simulink model "joint_space_trajectory_control_incomplete"  (R2022b)
settings: Solver=FixedStepDiscrete  StartTime=0.0  StopTime=inf  FixedStep=0.001  RelTol=1e-3  EnableMultiTasking=on
PreLoadFcn:
  | demos_common_configs();
  | 
  | collision_behavior = ones(1,52)*100;
undefined symbols (not defined in the file): ddQ2_desired, ddQ4_desired, dQ2_desired, dQ4_desired, Q2_desired, Q4_desired, q_init, T
libraries: franka_simulink_library_misc x5, franka_simulink_library x3
settings Model: SimulationMode=external  ExtModeTrigDuration=10000  Creator=vasi_ko  LastModifiedBy=s2ajami
settings SolverCC: AlgebraicLoopSolver=TrustRegion
settings DataIOCC: LimitDataPoints=on  SaveFormat=Array  ReturnWorkspaceOutputs=off
settings OptimizationCC: EnhancedBackFolding=on  PassReuseOutputArgsAs=Individual arguments  ZeroExternalMemoryAtStartup=off  ZeroInternalMemoryAtStartup=off  OptimizeBlockOrder=speed  DifferentSizesBufferReuse=on  OptimizationCustomize=off  EfficientTunableParamExpr=on
settings DebuggingCC: SolverPrmCheckMsg=warning  ParameterTunabilityLossMsg=error  UnconnectedInputMsg=warning  UnconnectedOutputMsg=warning  UnconnectedLineMsg=warning  SFUnexpectedBacktrackingDiag=warning  SFNoUnconditionalDefaultTransitionDiag=warning  SFExecutionAtInitializationDiag=none  SFMachineParentedDataDiag=warning  ArithmeticOperatorsInVariantConditions=warning
settings HardwareCC: ProdBitPerLong=64  ProdHWDeviceType=Intel->x86-64 (Linux 64)  TargetBitPerPointer=64  TargetBitPerSizeT=64  TargetBitPerPtrDiffT=64  TargetLongLongMode=on  TargetIntDivRoundTo=Zero  TargetEndianess=LittleEndian  TargetWordSize=64  TargetHWDeviceType=MATLAB Host
settings ModelReferenceCC: EnableRefExpFcnMdlSchedulingChecks=on  PropagateSignalLabelsOutOfModel=off
settings SFSimCC: SimUseLocalCustomCode=off  MATLABDynamicMemAlloc=off  CustomCodeUndefinedFunction=UseInterfaceOnly  SimTargetLang=C++
settings RTWCC: Description=Embedded Coder  SystemTargetFile=franka_emika_panda.tlc  GenCodeOnly=on  TemplateMakefile=ert_default_tmf  RTWVerbose=off  RTWUseLocalCustomCode=off  Toolchain=Franka Simulink | gmake (64-bit linux)  BuildConfiguration=Faster Runs  TargetLang=C++  DLArmComputeVersion=19.05
settings CodeAppCC: ForceParamTrailComments=on  IgnoreCustomStorageClasses=off  OperatorAnnotations=on  SimulinkDataObjDesc=on  SFDataObjDesc=on  InsertBlockDesc=on
settings STFCustomTargetCC: TargetLangStandard=C99 (ISO)  MultiwordLength=256  GenerateSampleERTMain=on  ModelReferenceCompliant=off  CombineOutputUpdateFcns=on  ERTCustomFileBanners=on  SupportNonInlinedSFcns=off  RemoveResetFunc=on  MATLABClassNameForMDSCustomization=Simulink.SoftwareTarget.ERTCustomization  CPPClassGenCompliant=on  UseToolchainInfoCompliant=on  SystemTargetFile=franka_emika_panda.tlc
settings ERTTargetCC: TargetLangStandard=C99 (ISO)  GenerateSampleERTMain=on  ModelReferenceCompliant=off  ParMdlRefBuildCompliant=off  CompOptLevelCompliant=off  ConcurrentExecutionCompliant=off  SupportContinuousTime=on  ModelStepFunctionPrototypeControlCompliant=off  ExtMode=on  ExtModeMexArgs='129.97.71.26' 0 17725  ERTCustomFileTemplate=franka_emika_panda_file_process.tlc
settings ConfigComp: CovMetricSettings=dw  CovSaveCumulativeToWorkspaceVar=on  CovSaveSingleToWorkspaceVar=on  CovExternalEMLEnable=off  CovSFcnEnable=off

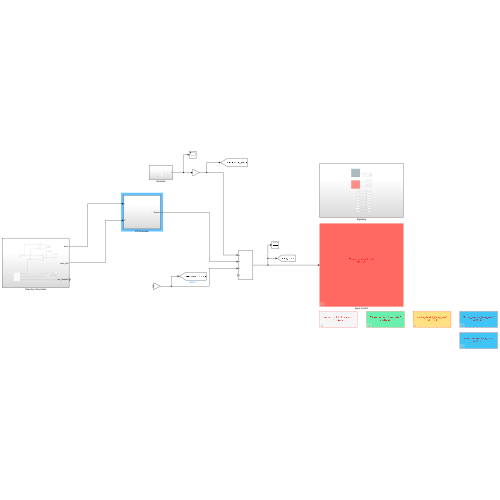
[thumbnail: Simulink's stored preview of the top-level diagram]
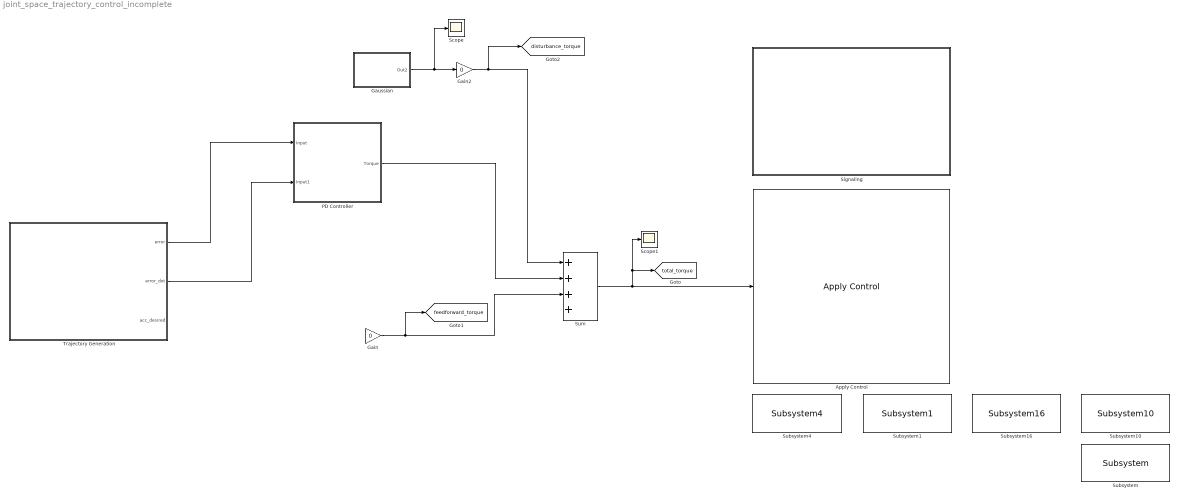
== system joint_space_trajectory_control_incomplete ==
  Apply Control : franka_simulink_library/Apply Control  robot_ip=robot_ip  gripper_attached=off  control_mode=Torque Control  controller_choice=Joint Impedance Controller  elbow_control=on  collision_thresholds=100*ones(1,52)  joint_impedance=joint_impedance  cartesian_impedance=cartesian_impedance  load_inertia=load_inertia  EE_T_K=EE_T_K  init_joint_configuration_req=on  init_joint_configuration=[0, -pi/4, 0, -3 * pi/4, 0, pi/2, pi/4]
  Gain : Gain  Gain=0
  Gain2 : Gain  Gain=0
  Gaussian : Subsystem
  PD Controller : Subsystem
  Scope : Scope
  Scope1 : Scope
  Signaling : Subsystem
  Subsystem : franka_simulink_library_misc/Subsystem  SystemSampleTime=-1  VariantActivationTime=update diagram  Latency=0  AutoFrameSizeCalculation=off
  Subsystem1 : franka_simulink_library_misc/Subsystem1  SystemSampleTime=-1  VariantActivationTime=update diagram  Latency=0  AutoFrameSizeCalculation=off
  Subsystem10 : franka_simulink_library_misc/Subsystem10  SystemSampleTime=-1  VariantActivationTime=update diagram  Latency=0  AutoFrameSizeCalculation=off
  Subsystem16 : franka_simulink_library_misc/Subsystem16  SystemSampleTime=-1  VariantActivationTime=update diagram  Latency=0  AutoFrameSizeCalculation=off
  Subsystem4 : franka_simulink_library_misc/Subsystem4  SystemSampleTime=-1  VariantActivationTime=update diagram  Latency=0  AutoFrameSizeCalculation=off
  Sum : Sum  Inputs=++++
  Trajectory Generation : Subsystem
  tag scope: disturbance_torque=global, feedforward_torque=global, total_torque=global
  wires:
  Sum/1 -> Scope1/1, [total_torque], Apply Control/1
  Trajectory Generation/1(error) -> PD Controller/1(Input)
  Trajectory Generation/2(error_dot) -> PD Controller/2(Input1)
  PD Controller/1(Torque) -> Sum/2
  Gain/1 -> [feedforward_torque], Sum/3
  Gain2/1 -> [disturbance_torque], Sum/1
  Gaussian/1(Out2) -> Scope/1, Gain2/1

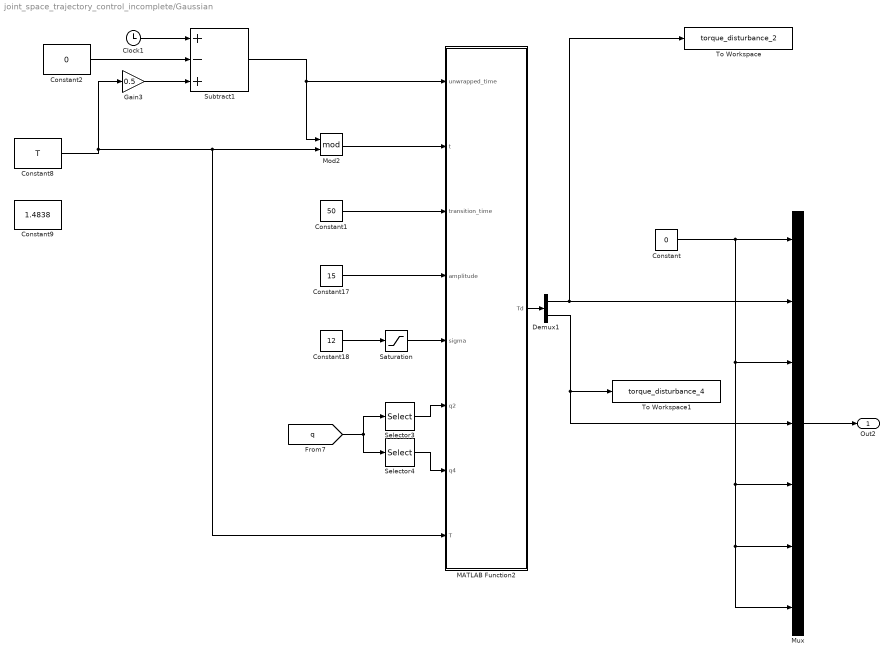
== system joint_space_trajectory_control_incomplete/Gaussian ==
  Clock1 : Clock
  Constant : Constant  Value=0
  Constant1 : Constant  Value=50
  Constant17 : Constant  Value=15
  Constant18 : Constant  Value=12
  Constant2 : Constant  Value=0
  Constant8 : Constant  Value=T
  Constant9 : Constant  Value=1.4838
  Demux1 : Demux  Outputs=2
  Gain3 : Gain  Gain=0.5
  MATLAB Function2 : MATLAB Function  TreatAsAtomicUnit=on
  Mod2 : Math  Operator=mod
  Mux : Mux  Inputs=7
  Saturation : Saturate  UpperLimit=inf  LowerLimit=12
  Selector3 : Selector  InputPortWidth=7  IndexOptions=Index vector (dialog)  Indices=[2]  OutputSizes=1
  Selector4 : Selector  InputPortWidth=7  IndexOptions=Index vector (dialog)  Indices=[4]  OutputSizes=1
  Subtract1 : Sum  Inputs=+-+
  To Workspace : ToWorkspace  VariableName=torque_disturbance_2  SaveFormat=Structure With Time  SampleTime=-1
  To Workspace1 : ToWorkspace  VariableName=torque_disturbance_4  SaveFormat=Structure With Time  SampleTime=-1
  Out2 : Outport
  wires:
  Mux/1 -> Out2/1
  Constant/1 -> Mux/3, Mux/5, Mux/6, Mux/7, Mux/1
  Gain3/1 -> Subtract1/3
  Constant17/1 -> MATLAB Function2/4(amplitude)
  Constant18/1 -> Saturation/1
  Saturation/1 -> MATLAB Function2/5(sigma)
  Clock1/1 -> Subtract1/1
  MATLAB Function2/1(Td) -> Demux1/1
  Demux1/1 -> Mux/2, To Workspace/1
  Demux1/2 -> Mux/4, To Workspace1/1
  Constant8/1 -> MATLAB Function2/8(T), Mod2/2, Gain3/1
  Mod2/1 -> MATLAB Function2/2(t)
  Subtract1/1 -> MATLAB Function2/1(unwrapped_time), Mod2/1
  Constant1/1 -> MATLAB Function2/3(transition_time)
  Constant2/1 -> Subtract1/2
  Selector3/1 -> MATLAB Function2/6(q2)
  Selector4/1 -> MATLAB Function2/7(q4)
  [q] -> Selector3/1, Selector4/1

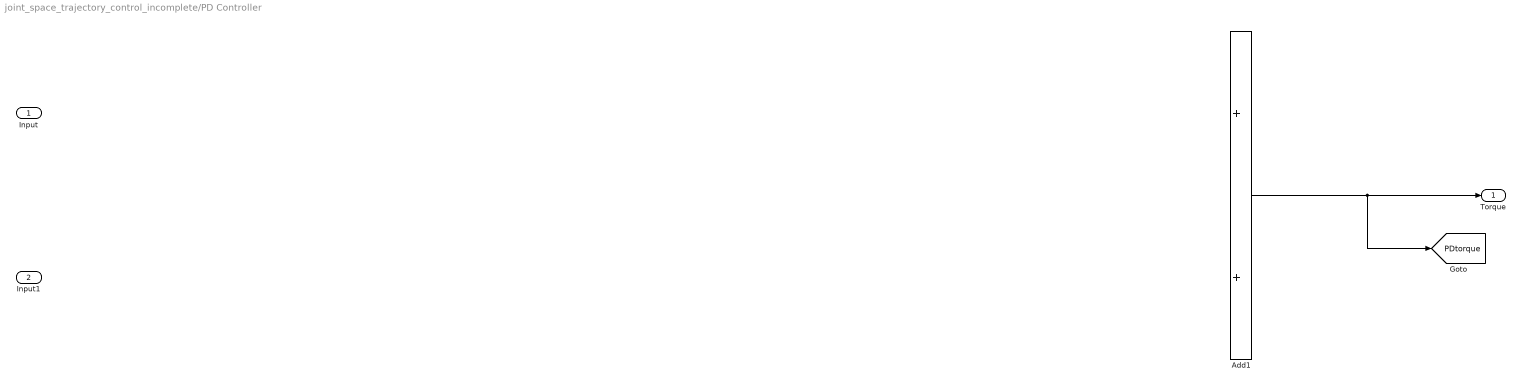
== system joint_space_trajectory_control_incomplete/PD Controller ==
  Input : Inport
  Input1 : Inport  Port=2
  Add1 : Sum
  Torque : Outport
  tag scope: PDtorque=global
  wires:
  Add1/1 -> [PDtorque], Torque/1

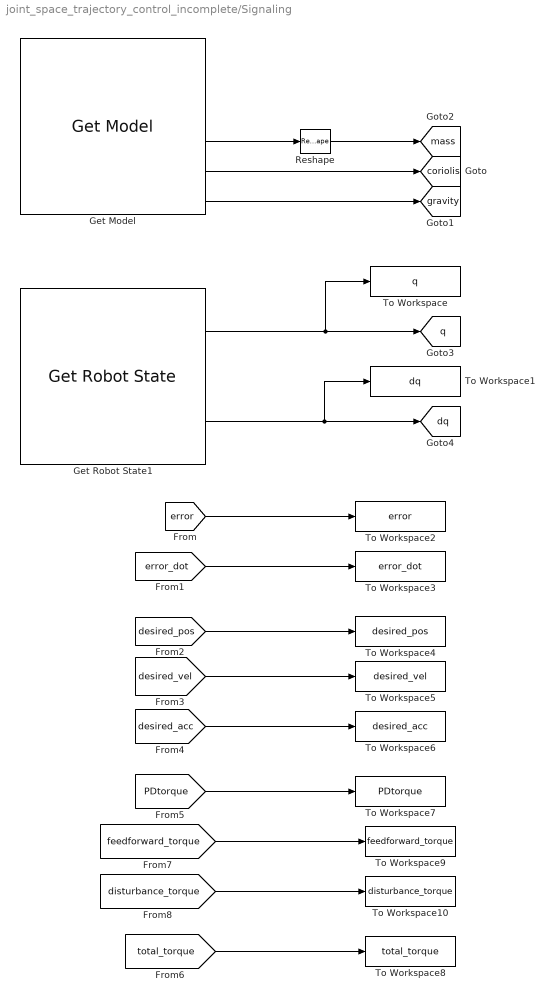
== system joint_space_trajectory_control_incomplete/Signaling ==
  Get Model : franka_simulink_library/Get Model  robot_ip=robot_ip
  Get Robot State1 : franka_simulink_library/Get Robot State  robot_ip=robot_ip  signals_requested='q dq'
  Reshape : Reshape  OutputDimensionality=Customize  OutputDimensions=[7,7]
  To Workspace : ToWorkspace  VariableName=q  SaveFormat=Structure With Time  SampleTime=-1
  To Workspace1 : ToWorkspace  VariableName=dq  SaveFormat=Structure With Time  SampleTime=-1
  To Workspace10 : ToWorkspace  VariableName=disturbance_torque  SaveFormat=Structure With Time  SampleTime=-1
  To Workspace2 : ToWorkspace  VariableName=error  SaveFormat=Structure With Time  SampleTime=-1
  To Workspace3 : ToWorkspace  VariableName=error_dot  SaveFormat=Structure With Time  SampleTime=-1
  To Workspace4 : ToWorkspace  VariableName=desired_pos  SaveFormat=Structure With Time  SampleTime=-1
  To Workspace5 : ToWorkspace  VariableName=desired_vel  SaveFormat=Structure With Time  SampleTime=-1
  To Workspace6 : ToWorkspace  VariableName=desired_acc  SaveFormat=Structure With Time  SampleTime=-1
  To Workspace7 : ToWorkspace  VariableName=PDtorque  SaveFormat=Structure With Time  SampleTime=-1
  To Workspace8 : ToWorkspace  VariableName=total_torque  SaveFormat=Structure With Time  SampleTime=-1
  To Workspace9 : ToWorkspace  VariableName=feedforward_torque  SaveFormat=Structure With Time  SampleTime=-1
  tag scope: coriolis=global, dq=global, gravity=global, mass=global, q=global
  wires:
  Get Model/5 -> [coriolis]
  Get Model/6 -> [gravity]
  Get Model/4 -> Reshape/1
  Get Robot State1/1 -> To Workspace/1, [q]
  Get Robot State1/2 -> To Workspace1/1, [dq]
  [desired_acc] -> To Workspace6/1
  [desired_vel] -> To Workspace5/1
  [desired_pos] -> To Workspace4/1
  [error_dot] -> To Workspace3/1
  [error] -> To Workspace2/1
  [PDtorque] -> To Workspace7/1
  [total_torque] -> To Workspace8/1
  Reshape/1 -> [mass]
  [feedforward_torque] -> To Workspace9/1
  [disturbance_torque] -> To Workspace10/1

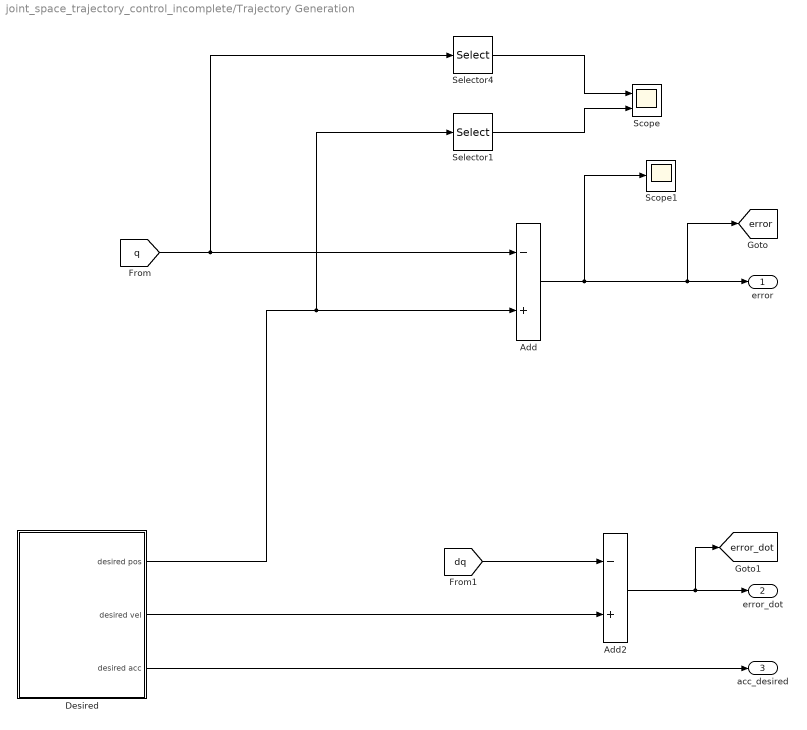
== system joint_space_trajectory_control_incomplete/Trajectory Generation ==
  Add : Sum  Inputs=-+
  Add2 : Sum  Inputs=-+
  Desired : Subsystem
  Scope : Scope  NumInputPorts=2
  Scope1 : Scope
  Selector1 : Selector  InputPortWidth=7  IndexOptions=Index vector (dialog)  Indices=[6]  OutputSizes=1
  Selector4 : Selector  InputPortWidth=7  IndexOptions=Index vector (dialog)  Indices=[6]  OutputSizes=1
  error : Outport
  error_dot : Outport  Port=2
  acc_desired : Outport  Port=3
  tag scope: error=global, error_dot=global
  wires:
  Desired/2(desired vel) -> Add2/2
  Desired/1(desired pos) -> Selector1/1, Add/2
  Add/1 -> Scope1/1, error/1, [error]
  Add2/1 -> [error_dot], error_dot/1
  Desired/3(desired acc) -> acc_desired/1
  [dq] -> Add2/1
  Selector4/1 -> Scope/1
  Selector1/1 -> Scope/2
  [q] -> Selector4/1, Add/1

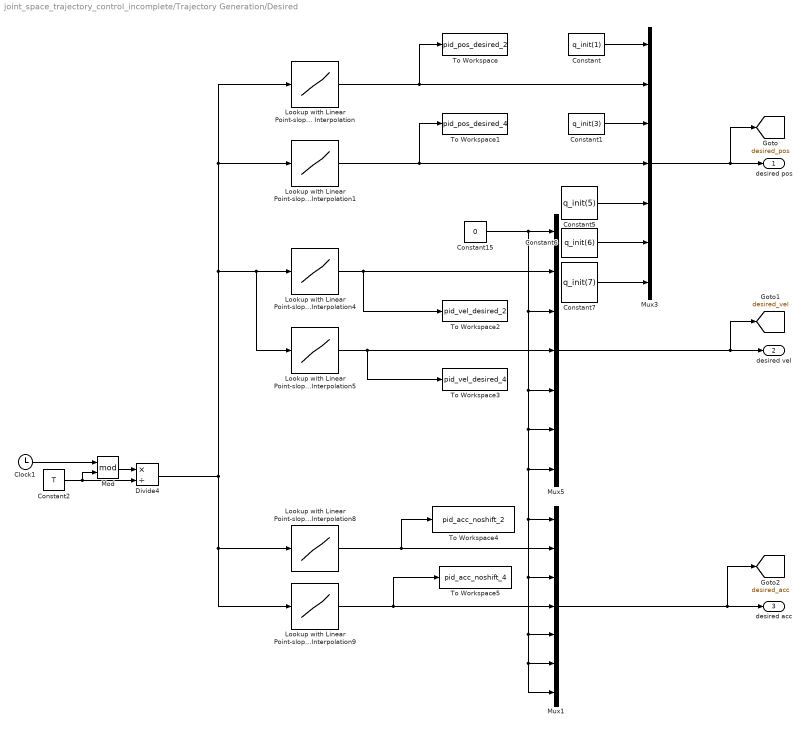
== system joint_space_trajectory_control_incomplete/Trajectory Generation/Desired ==
  Clock1 : Clock
  Constant : Constant  Value=q_init(1)
  Constant1 : Constant  Value=q_init(3)
  Constant15 : Constant  Value=0
  Constant2 : Constant  Value=T
  Constant5 : Constant  Value=q_init(5)
  Constant6 : Constant  Value=q_init(6)
  Constant7 : Constant  Value=q_init(7)
  Divide4 : Product  Inputs=*/
  Lookup with Linear Point-slope Interpolation : Lookup_n-D  NumberOfTableDimensions=1  BreakpointsForDimension1=linspace(0,1,length(Q2_desired))  Table=Q2_desired  InternalRulePriority=Speed  RndMeth=Simplest
  Lookup with Linear Point-slope Interpolation1 : Lookup_n-D  NumberOfTableDimensions=1  BreakpointsForDimension1=linspace(0,1,length(Q4_desired))  Table=Q4_desired  InternalRulePriority=Speed  RndMeth=Simplest
  Lookup with Linear Point-slope Interpolation4 : Lookup_n-D  NumberOfTableDimensions=1  BreakpointsForDimension1=linspace(0,1,length(dQ2_desired))  Table=dQ2_desired  InternalRulePriority=Speed  RndMeth=Simplest
  Lookup with Linear Point-slope Interpolation5 : Lookup_n-D  NumberOfTableDimensions=1  BreakpointsForDimension1=linspace(0,1,length(dQ4_desired))  Table=dQ4_desired  InternalRulePriority=Speed  RndMeth=Simplest
  Lookup with Linear Point-slope Interpolation8 : Lookup_n-D  NumberOfTableDimensions=1  BreakpointsForDimension1=linspace(0,1,length(ddQ2_desired))  Table=ddQ2_desired  InternalRulePriority=Speed  RndMeth=Simplest
  Lookup with Linear Point-slope Interpolation9 : Lookup_n-D  NumberOfTableDimensions=1  BreakpointsForDimension1=linspace(0,1,length(ddQ2_desired))  Table=ddQ4_desired  InternalRulePriority=Speed  RndMeth=Simplest
  Mod : Math  Operator=mod
  Mux1 : Mux  Inputs=7
  Mux3 : Mux  Inputs=7
  Mux5 : Mux  Inputs=7
  To Workspace : ToWorkspace  VariableName=pid_pos_desired_2  SaveFormat=Structure With Time  SampleTime=-1
  To Workspace1 : ToWorkspace  VariableName=pid_pos_desired_4  SaveFormat=Structure With Time  SampleTime=-1
  To Workspace2 : ToWorkspace  VariableName=pid_vel_desired_2  SaveFormat=Structure With Time  SampleTime=-1
  To Workspace3 : ToWorkspace  VariableName=pid_vel_desired_4  SaveFormat=Structure With Time  SampleTime=-1
  To Workspace4 : ToWorkspace  VariableName=pid_acc_noshift_2  SaveFormat=Structure With Time  SampleTime=-1
  To Workspace5 : ToWorkspace  VariableName=pid_acc_noshift_4  SaveFormat=Structure With Time  SampleTime=-1
  desired pos : Outport
  desired vel : Outport  Port=2
  desired acc : Outport  Port=3
  tag scope: desired_acc=global, desired_pos=global, desired_vel=global
  wires:
  Lookup with Linear Point-slope Interpolation4/1 -> Mux5/2, To Workspace2/1
  Constant15/1 -> Mux5/3, Mux5/5, Mux5/6, Mux5/7, Mux1/7, Mux1/6, Mux1/5, Mux1/3, Mux1/1, Mux5/1
  Clock1/1 -> Mod/1
  Lookup with Linear Point-slope Interpolation1/1 -> Mux3/4, To Workspace1/1
  Mux5/1 -> [desired_vel], desired vel/1
  Lookup with Linear Point-slope Interpolation8/1 -> To Workspace4/1, Mux1/2
  Mux1/1 -> [desired_acc], desired acc/1
  Lookup with Linear Point-slope Interpolation/1 -> Mux3/2, To Workspace/1
  Lookup with Linear Point-slope Interpolation5/1 -> Mux5/4, To Workspace3/1
  Constant6/1 -> Mux3/6
  Constant5/1 -> Mux3/5
  Constant1/1 -> Mux3/3
  Divide4/1 -> Lookup with Linear Point-slope Interpolation/1, Lookup with Linear Point-slope Interpolation1/1, Lookup with Linear Point-slope Interpolation5/1, Lookup with Linear Point-slope Interpolation4/1, Lookup with Linear Point-slope Interpolation9/1, Lookup with Linear Point-slope Interpolation8/1
  Constant7/1 -> Mux3/7
  Lookup with Linear Point-slope Interpolation9/1 -> To Workspace5/1, Mux1/4
  Constant/1 -> Mux3/1
  Mux3/1 -> [desired_pos], desired pos/1
  Constant2/1 -> Mod/2, Divide4/2
  Mod/1 -> Divide4/1

== matlab function joint_space_trajectory_control_incomplete/Gaussian/MATLAB Function2 ==
  data: unwrapped_time input; t input; transition_time input; amplitude input; sigma input; Td output; q2 input; q4 input; T input
function Td = gaussian_generator(unwrapped_time, t,transition_time, amplitude, sigma, q2, q4, T)
    gain = 0;
    l1 = sqrt(0.316^2 + 0.088^2);
    l2 = sqrt(0.384^2 + 0.088^2);
    persistent enable
    if isempty(enable)
        enable = 0;
    end
    
    if unwrapped_time > T
        enable = 1;
        gain = amplitude*(unwrapped_time - T)/(transition_time);
    end
    
    if gain > amplitude
        gain = amplitude;
    end
    f = gain * exp(-sigma*(t-T/2)^2)*enable;
    F = [1; 0].*f ;
    J = [-l1*cos(q2)-l2*cos(q2-q4) l2*cos(q2-q4);...
         -l1*sin(q2)-l2*sin(q2-q4) l2*sin(q2-q4)];

    % Disturbance Torque
    Td = J'*F *enable;
end
